simulink model "AOO_VOO_VVI_AAI_v4"  (R2025a)
settings: Solver=FixedStepAuto  StartTime=0.0  StopTime=10.0  FixedStep=1e-3  RelTol=1e-3  EnableMultiTasking=on
undefined symbols (not defined in the file or in its folder): D0, D1, D10, D11, D12, D13, D2, D3, D4, D5, D6, D7, D8, D9, PTA0, PTA1, PTA2, PTB23, PTB9, PTC16, PTC17, PTC2, PTC3, PTC4, PTD0, PTD1, PTD2, PTD3
libraries: frdmk64flib x16
settings Model: SimulationMode=external  ExtModeTrigDuration=5  Creator=emily  LastModifiedBy=tphil
settings SolverCC: AlgebraicLoopSolver=TrustRegion
settings OptimizationCC: EnhancedBackFolding=on  PassReuseOutputArgsAs=Individual arguments  ZeroExternalMemoryAtStartup=off  ZeroInternalMemoryAtStartup=off  MaxStackSize=64  OptimizeBlockOrder=speed  DifferentSizesBufferReuse=on  OptimizationCustomize=off  EfficientTunableParamExpr=on
settings DebuggingCC: ParameterTunabilityLossMsg=error  UnconnectedInputMsg=warning  UnconnectedOutputMsg=warning  UnconnectedLineMsg=warning
settings HardwareCC: ProdBitPerPointer=32.0  ProdBitPerSizeT=32.0  ProdBitPerPtrDiffT=32.0  ProdLargestAtomicInteger=Long  ProdLargestAtomicFloat=Double  ProdWordSize=32.0  ProdHWDeviceType=ARM Compatible->ARM Cortex
settings ModelReferenceCC: EnableRefExpFcnMdlSchedulingChecks=on
settings SFSimCC: MATLABDynamicMemAlloc=off
settings RTWCC: SystemTargetFile=ert.tlc  HardwareBoard=NXP FRDM-K64F  TLCOptions="-aInlineSetEventsForThisBaseRateFcn=TLC_FALSE -aSuppressMultiTaskScheduler=TLC_FALSE  -aRateBasedStepFcn=0"  TemplateMakefile=ert_default_tmf  Toolchain=GNU Tools for ARM Embedded Processors  GPUComputeCapability=3.5  Description=Embedded Coder
settings CodeAppCC: ForceParamTrailComments=on  IgnoreCustomStorageClasses=off  OperatorAnnotations=on  SimulinkDataObjDesc=on  SFDataObjDesc=on  InsertBlockDesc=on
settings ERTTargetCC: ExtModeTransport=0.0  ExtModeStaticAlloc=off  ExtModeMexFile=ext_comm  ExtModeIntrfLevel=Level1  InlinedParameterPlacement=Hierarchical  DynamicArrayContainerType=coder::array

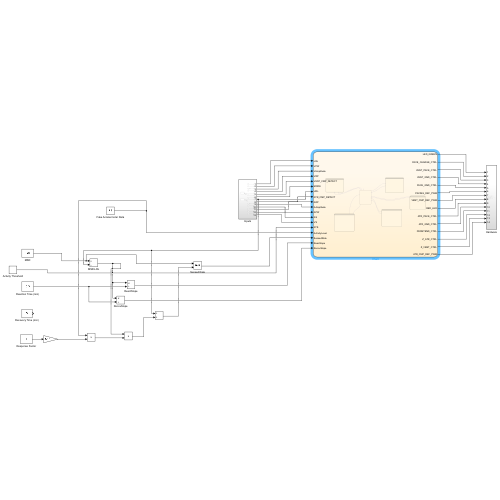
[thumbnail: Simulink's stored preview of the top-level diagram]
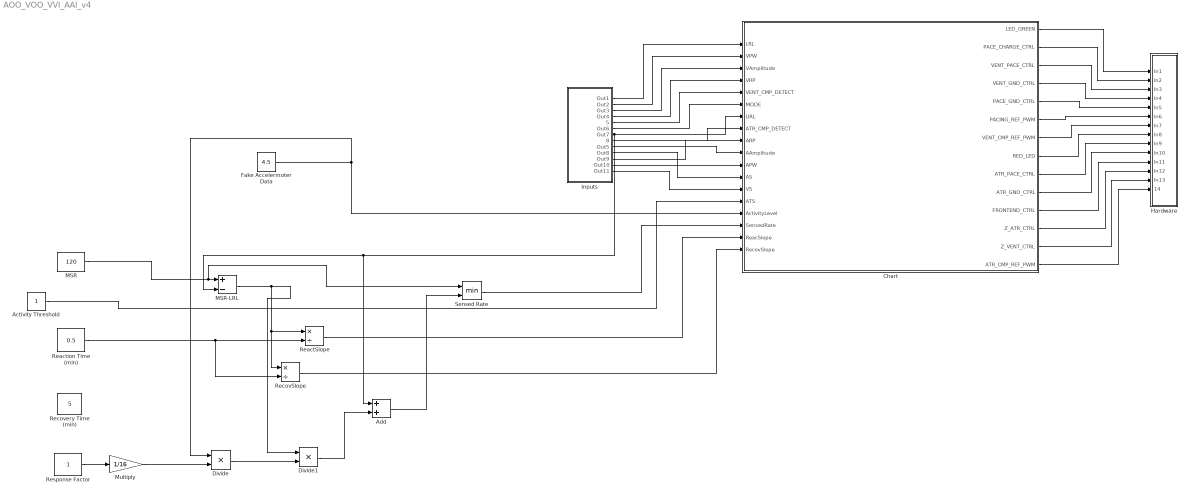
== system AOO_VOO_VVI_AAI_v4 ==
  Activity Threshold : Constant
  Add : Sum
  Chart : Stateflow chart  TreatAsAtomicUnit=on
  Divide : Product  Inputs=**
  Divide1 : Product  Inputs=**
  Fake Accelermoter Data : Constant  Value=4.5
  Hardware : Subsystem
  Inputs : Subsystem
  MSR : Constant  Value=120
  MSR-LRL : Sum  Inputs=+-
  Multiply : Gain  Gain=1/16
  ReactSlope : Product  Inputs=*/
  Reaction Time (min) : Constant  Value=0.5
  RecovSlope : Product  Inputs=*/
  Recovery Time (min) : Constant  Value=5
  Response Factor : Constant
  Sensed Rate : MinMax  Inputs=2
  wires:
  Chart/2(PACE_CHARGE_CTRL) -> Hardware/2(In2)
  Chart/4(VENT_GND_CTRL) -> Hardware/4(In4)
  Chart/12(Z_ATR_CTRL) -> Hardware/12(In12)
  Inputs/4(Out4) -> Chart/4(VRP)
  Chart/7(VENT_CMP_REF_PWM) -> Hardware/7(In7)
  Inputs/5(5) -> Chart/5(VENT_CMP_DETECT)
  Inputs/3(Out3) -> Chart/3(VAmplitude)
  Chart/3(VENT_PACE_CTRL) -> Hardware/3(In3)
  Inputs/6(Out6) -> Chart/6(MODE)
  Inputs/1(Out1) -> Chart/1(LRL)
  Chart/6(PACING_REF_PWM) -> Hardware/6(In6)
  Chart/13(Z_VENT_CTRL) -> Hardware/13(In13)
  Chart/9(ATR_PACE_CTRL) -> Hardware/9(In9)
  Chart/11(FRONTEND_CTRL) -> Hardware/11(In11)
  Chart/8(RED_LED) -> Hardware/8(In8)
  Chart/10(ATR_GND_CTRL) -> Hardware/10(In10)
  Inputs/2(Out2) -> Chart/2(VPW)
  Chart/5(PACE_GND_CTRL) -> Hardware/5(In5)
  Chart/1(LED_GREEN) -> Hardware/1(In1)
  Inputs/7(Out7) -> Add/1, MSR-LRL/2, Chart/7(URL)
  Inputs/8(8) -> Chart/8(ATR_CMP_DETECT)
  Chart/14(ATR_CMP_REF_PWM) -> Hardware/14(14)
  Inputs/9(Out5) -> Chart/10(AAmplitude)
  Inputs/10(Out8) -> Chart/11(APW)
  Inputs/11(Out9) -> Chart/9(ARP)
  Inputs/12(Out10) -> Chart/12(AS)
  Inputs/13(Out11) -> Chart/13(VS)
  MSR/1 -> Sensed Rate/1, MSR-LRL/1
  MSR-LRL/1 -> RecovSlope/1, ReactSlope/1, Divide1/1
  Reaction Time (min)/1 -> RecovSlope/2, ReactSlope/2
  Response Factor/1 -> Multiply/1
  Multiply/1 -> Divide/2
  Divide/1 -> Divide1/2
  Divide1/1 -> Add/2
  Add/1 -> Sensed Rate/2
  Sensed Rate/1 -> Chart/16(SensedRate)
  Activity Threshold/1 -> Chart/14(ATS)
  ReactSlope/1 -> Chart/17(ReacSlope)
  RecovSlope/1 -> Chart/18(RecovSlope)
  Fake Accelermoter Data/1 -> Divide/1, Chart/15(ActivityLevel)

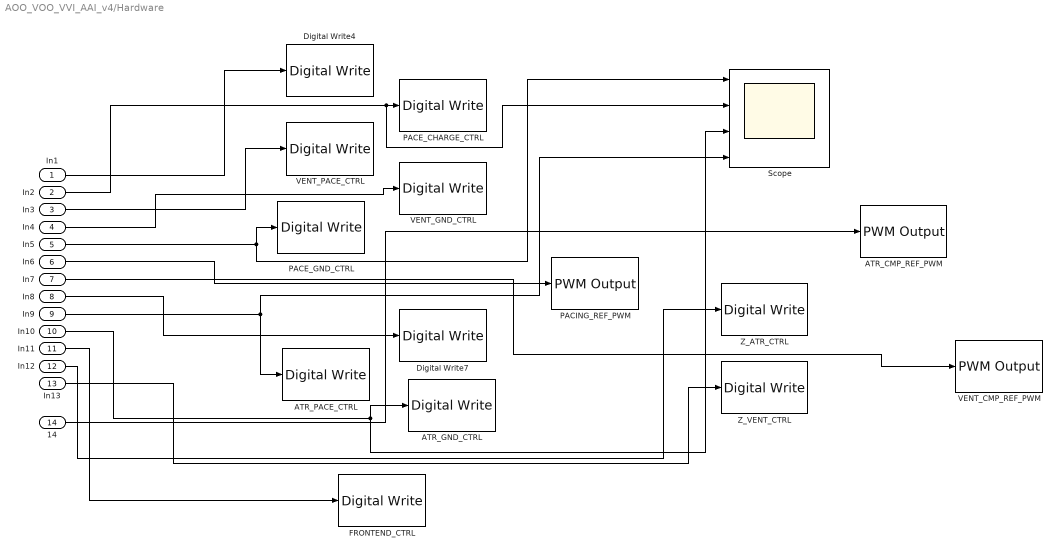
== system AOO_VOO_VVI_AAI_v4/Hardware ==
  In1 : Inport
  In2 : Inport  Port=2
  In3 : Inport  Port=3
  In4 : Inport  Port=4
  In5 : Inport  Port=5
  In6 : Inport  Port=6
  In7 : Inport  Port=7
  In8 : Inport  Port=8
  In9 : Inport  Port=9
  In10 : Inport  Port=10
  In11 : Inport  Port=11
  In12 : Inport  Port=12
  In13 : Inport  Port=13
  14 : Inport  Port=14
  ATR_CMP_REF_PWM : frdmk64flib/PWM Output  Whichpin=PTC2 (D6)  InitialFrequency=2000  InitialDutyCycle=0
  ATR_GND_CTRL : frdmk64flib/Digital Write  Whichpin=PTD2 (D11)
  ATR_PACE_CTRL : frdmk64flib/Digital Write  Whichpin=PTA0 (D8)
  Digital Write4 : frdmk64flib/Digital Write  Whichpin=GREEN_LED
  Digital Write7 : frdmk64flib/Digital Write  Whichpin=RED_LED
  FRONTEND_CTRL : frdmk64flib/Digital Write  Whichpin=PTD1 (D13)
  PACE_CHARGE_CTRL : frdmk64flib/Digital Write  Whichpin=PTB9 (D2)
  PACE_GND_CTRL : frdmk64flib/Digital Write  Whichpin=PTD0 (D10)
  PACING_REF_PWM : frdmk64flib/PWM Output  Whichpin=PTA2 (D5)  InitialFrequency=2000  InitialDutyCycle=30
  Scope : Scope  NumInputPorts=4
      settings: DataLoggingVariableName=ScopeData2
  VENT_CMP_REF_PWM : frdmk64flib/PWM Output  Whichpin=PTA1 (D3)  InitialFrequency=2000  InitialDutyCycle=0
  VENT_GND_CTRL : frdmk64flib/Digital Write  Whichpin=PTD3 (D12)
  VENT_PACE_CTRL : frdmk64flib/Digital Write  Whichpin=PTC4 (D9)
  Z_ATR_CTRL : frdmk64flib/Digital Write  Whichpin=PTB23 (D4)
  Z_VENT_CTRL : frdmk64flib/Digital Write  Whichpin=PTC3 (D7)
  wires:
  In10/1 -> Scope/3, ATR_GND_CTRL/1
  In2/1 -> Scope/2, PACE_CHARGE_CTRL/1
  In6/1 -> PACING_REF_PWM/1
  In4/1 -> VENT_GND_CTRL/1
  In13/1 -> Z_VENT_CTRL/1
  In1/1 -> Digital Write4/1
  In5/1 -> PACE_GND_CTRL/1, Scope/1
  In3/1 -> VENT_PACE_CTRL/1
  In9/1 -> ATR_PACE_CTRL/1, Scope/4
  In8/1 -> Digital Write7/1
  In12/1 -> Z_ATR_CTRL/1
  In11/1 -> FRONTEND_CTRL/1
  14/1 -> ATR_CMP_REF_PWM/1
  In7/1 -> VENT_CMP_REF_PWM/1

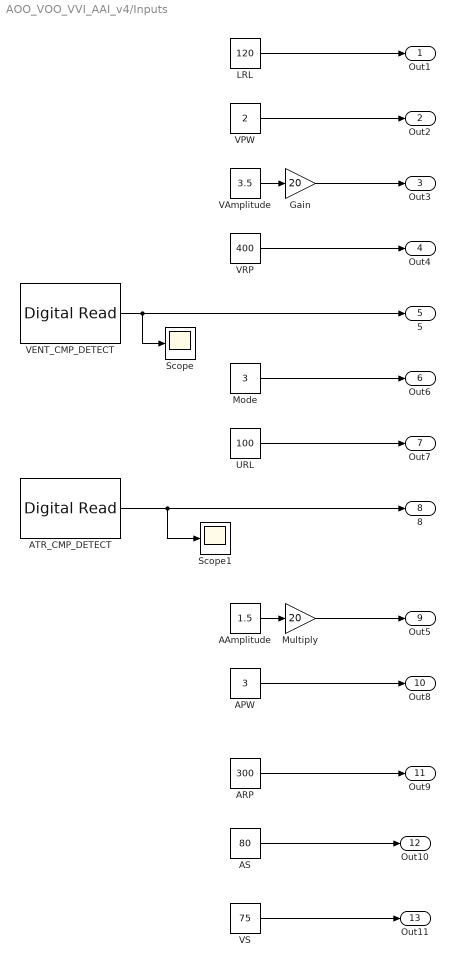
== system AOO_VOO_VVI_AAI_v4/Inputs ==
  AAmplitude : Constant  Value=1.5  OutDataTypeStr=double
  APW : Constant  Value=3  OutDataTypeStr=double
  ARP : Constant  Value=300  OutDataTypeStr=double
  AS : Constant  Value=80  OutDataTypeStr=double
  ATR_CMP_DETECT : frdmk64flib/Digital Read  Whichpin=PTC16 (D0)  SampleTime=-1
  Gain : Gain  Gain=20
  LRL : Constant  Value=120  OutDataTypeStr=double
  Mode : Constant  Value=3  OutDataTypeStr=int16
  Multiply : Gain  Gain=20
  Scope : Scope
      settings: ActiveDisplayYMinimum=0.9  ActiveDisplayYMaximum=1.1
  Scope1 : Scope
      settings: ActiveDisplayYMinimum=0.9  ActiveDisplayYMaximum=1.1
  URL : Constant  Value=100  OutDataTypeStr=double
  VAmplitude : Constant  Value=3.5  OutDataTypeStr=double
  VENT_CMP_DETECT : frdmk64flib/Digital Read  Whichpin=PTC17 (D1)  SampleTime=inf
  VPW : Constant  Value=2  OutDataTypeStr=double
  VRP : Constant  Value=400  OutDataTypeStr=double
  VS : Constant  Value=75  OutDataTypeStr=double
  Out1 : Outport
  Out2 : Outport  Port=2
  Out3 : Outport  Port=3
  Out4 : Outport  Port=4
  5 : Outport  Port=5
  Out6 : Outport  Port=6
  Out7 : Outport  Port=7
  8 : Outport  Port=8
  Out5 : Outport  Port=9
  Out8 : Outport  Port=10
  Out9 : Outport  Port=11
  Out10 : Outport  Port=12
  Out11 : Outport  Port=13
  wires:
  VPW/1 -> Out2/1
  VAmplitude/1 -> Gain/1
  VENT_CMP_DETECT/1 -> 5/1, Scope/1
  VRP/1 -> Out4/1
  Mode/1 -> Out6/1
  LRL/1 -> Out1/1
  Gain/1 -> Out3/1
  URL/1 -> Out7/1
  ATR_CMP_DETECT/1 -> Scope1/1, 8/1
  AAmplitude/1 -> Multiply/1
  Multiply/1 -> Out5/1
  APW/1 -> Out8/1
  ARP/1 -> Out9/1
  AS/1 -> Out10/1
  VS/1 -> Out11/1

== stateflow chart AOO_VOO_VVI_AAI_v4/Chart ==
  state VOO
    entry:
    % Initialize PACE_GND_CTRL and set the PWM amplitude to the Ventricular Amplitude
    PACE_GND_CTRL = 1;
    PACING_REF_PWM = VAmplitude;
    state TIMING
      entry:
      % upon entry into VOO send no pulse
      % and wait for a period - the VPW
      LED_GREEN = 0;
      VENT_PACE_CTRL = 0;
      PACE_CHARGE_CTRL =1;
      VENT_GND_CTRL = 1;
    state PULSE
      entry:
      % upon entry into VOO send no pulse
      % and wait for a period - the VPW
      LED_GREEN = 1;
      PACE_CHARGE_CTRL =0;
      VENT_PACE_CTRL = 1;
      VENT_GND_CTRL = 0;
    (default) -> VOO.TIMING
    VOO.PULSE -> VOO.TIMING : after(VPW, msec)
    VOO.TIMING -> VOO.PULSE : after(60000/LRL -VPW, msec)
  state AOO
    entry:
    % Initialize PACE_GND_CTRL and set the PWM amplitude to the Atrial Amplitude
    PACE_GND_CTRL = 1;
    PACING_REF_PWM = VAmplitude;
    state TIMING
      entry:
      % upon entry into AOO send no pulse
      % and wait for a period - the APW
      LED_GREEN = 0;
      ATR_PACE_CTRL = 0;
      PACE_CHARGE_CTRL =1;
      ATR_GND_CTRL = 1;
    state PULSE
      entry:
      % after set duration has passed, send
      % a pulse for the APW duration
      LED_GREEN = 1;
      PACE_CHARGE_CTRL =0;
      ATR_GND_CTRL = 0;
      ATR_PACE_CTRL = 1;
    (default) -> AOO.TIMING
    AOO.TIMING -> AOO.PULSE : after(60000/LRL -APW, msec)
    AOO.PULSE -> AOO.TIMING : after(APW, msec)
  state INITIALIZE
    entry:
    % Initialize inputs
    PACE_CHARGE_CTRL = 0;
    ATR_PACE_CTRL = 0;
    VENT_PACE_CTRL = 0;
    PACE_GND_CTRL = 1;
    ATR_GND_CTRL = 0;
    VENT_GND_CTRL=0;
    FRONTEND_CTRL=1;
    Z_ATR_CTRL = 0;
    Z_VENT_CTRL=0;
  state VVIR
    entry:
    % set PACE_GND_CTRL to 1 and the PWM amplitude to Ventricular Amplitude
    PACE_GND_CTRL = 1;
    PACING_REF_PWM = VAmplitude;
    % Set the ATR_CMP_REF_PWM to Ventricular sensitivity
    VENT_CMP_REF_PWM=VS;
    HeartRate = LRL
    %actTime and noactTime needs to be in mins
    actTime = 0
    noactTime = 0
    state AtSensedRate
      entry:
      HeartRate = SensedRate
    state IncreaseHeartRate
      entry:
      HeartRate = HeartRate+ReacSlope*actTime
    state WAIT
      entry:
      entry:
      % upon entry wait for signal to be
      % sensed or duration of no pulse
      % to pass
      PACE_CHARGE_CTRL = 1;
      Z_VENT_CTRL=1;
      VENT_PACE_CTRL = 0;
      VENT_GND_CTRL =1;
      RED_LED = 0;
      LED_GREEN = 0;
    state DecreaseHeartRate
      entry:
      HeartRate=HeartRate-RecovSlope*noactTime
    state AtLRL
      entry:
      HeartRate = LRL
    state PACE
      entry:
      % if no signal was sensed send pulse
      PACE_CHARGE_CTRL = 0;
      Z_VENT_CTRL=0;
      VENT_PACE_CTRL = 1;
      VENT_GND_CTRL = 0;
      RED_LED = 0;
      LED_GREEN = 1;
    state REFRACTORY
      entry:
      % if signal was sensed or VPW duration passed
      % wait for VRP duration and go to WAIT state
      PACE_CHARGE_CTRL = 1;
      Z_VENT_CTRL=1;
      VENT_PACE_CTRL = 0;
      VENT_GND_CTRL = 1;
      RED_LED = 1;
      LED_GREEN = 0;
    AtSensedRate -> (junction 162)
    (junction 143) -> AtSensedRate [order 1] : [HeartRate+ReacSlope*actTime>=SensedRate]
    (default) -> VVIR.WAIT
    VVIR.WAIT -> (junction 143) [order 2] : [ActivityLevel - ATS > 0]
    (junction 143) -> IncreaseHeartRate [order 2] : [HeartRate+ReacSlope*actTime < SensedRate]
    IncreaseHeartRate -> (junction 162)
    (junction 162) -> VVIR.WAIT
    AtLRL -> (junction 162)
    DecreaseHeartRate -> (junction 162)
    VVIR.WAIT -> (junction 150) [order 4] : [ActivityLevel - ATS < 0]
    (junction 150) -> DecreaseHeartRate [order 1] : [HeartRate-RecovSlope*noactTime > LRL]
    (junction 150) -> AtLRL [order 2] : [HeartRate-RecovSlope*noactTime <= LRL]
    VVIR.WAIT -> VVIR.REFRACTORY [order 1] : [VENT_CMP_DETECT == 1]
    VVIR.REFRACTORY -> VVIR.WAIT : after(VRP,msec)
    VVIR.WAIT -> VVIR.PACE [order 3] : after(60000/HeartRate - (VPW+VRP), msec)
    VVIR.PACE -> VVIR.REFRACTORY : after(VPW, msec)
  state VVI
    entry:
    % set PACE_GND_CTRL to 1 and the PWM amplitude to Ventricular Amplitude
    PACE_GND_CTRL = 1;
    PACING_REF_PWM = VAmplitude;
    % Set the ATR_CMP_REF_PWM to Ventricular sensitivity
    VENT_CMP_REF_PWM=VS;
    state PACE
      entry:
      % if no signal was sensed send pulse
      PACE_CHARGE_CTRL = 0;
      Z_VENT_CTRL=0;
      VENT_PACE_CTRL = 1;
      VENT_GND_CTRL = 0;
      RED_LED = 0;
      LED_GREEN = 1;
    state WAIT
      entry:
      % upon entry wait for signal to be
      % sensed or duration of no pulse
      % to pass
      PACE_CHARGE_CTRL = 1;
      Z_VENT_CTRL=1;
      VENT_PACE_CTRL = 0;
      VENT_GND_CTRL =1;
      RED_LED = 0;
      LED_GREEN = 0;
    state REFRACTORY
      entry:
      % if signal was sensed or VPW duration passed
      % wait for VRP duration and go to WAIT state
      PACE_CHARGE_CTRL = 1;
      Z_VENT_CTRL=1;
      VENT_PACE_CTRL = 0;
      VENT_GND_CTRL = 1;
      RED_LED = 1;
      LED_GREEN = 0;
    (default) -> VVI.WAIT
    VVI.WAIT -> VVI.PACE [order 1] : after(60000/LRL -(VPW+VRP), msec)
    VVI.PACE -> VVI.REFRACTORY : after(VPW,msec)
    VVI.WAIT -> VVI.REFRACTORY [order 2] : [VENT_CMP_DETECT==1]
    VVI.REFRACTORY -> VVI.WAIT : after(VRP, msec)
  state AAI
    entry:
    % set PACE_GND_CTRL to 1 and the PWM amplitude to Atrial Amplitude
    PACE_GND_CTRL = 1;
    PACING_REF_PWM = AAmplitude;
    % Set the ATR_CMP_REF_PWM to Atrial sensitivity
    ATR_CMP_REF_PWM=AS;
    state PACE
      entry:
      % if no signal was sensed send pulse
      PACE_CHARGE_CTRL = 0;
      ATR_PACE_CTRL = 1;
      ATR_GND_CTRL = 0;
      RED_LED = 0;
      LED_GREEN = 1;
    state WAIT
      entry:
      % upon entry wait for signal to be
      % sensed or duration of no pulse
      % to pass
      PACE_CHARGE_CTRL = 1;
      ATR_PACE_CTRL = 0;
      ATR_GND_CTRL =1;
      RED_LED = 0;
      LED_GREEN = 0;
    state REFRACTORY
      entry:
      % if signal was sensed or APW duration passed
      % wait for ARP duration and go to WAIT state
      PACE_CHARGE_CTRL = 1;
      ATR_PACE_CTRL = 0;
      ATR_GND_CTRL = 1;
      RED_LED = 1;
      LED_GREEN = 0;
    (default) -> AAI.WAIT
    AAI.WAIT -> AAI.PACE [order 1] : after(60000/LRL -(APW+ARP), msec)
    AAI.WAIT -> AAI.REFRACTORY [order 2] : [ATR_CMP_DETECT==1]
    AAI.REFRACTORY -> AAI.WAIT : after(ARP, msec)
    AAI.PACE -> AAI.REFRACTORY : after(APW,msec)
  INITIALIZE -> VOO [order 2] : [MODE==2]
  VOO -> INITIALIZE : [MODE~=2]
  AOO -> INITIALIZE : [MODE~=1]
  INITIALIZE -> AOO [order 1] : [MODE==1]
  (default) -> INITIALIZE
  AAI -> INITIALIZE : [MODE~=4]
  INITIALIZE -> VVIR [order 3] : [MODE==5]
  VVIR -> INITIALIZE : [MODE~=5]
  INITIALIZE -> VVI [order 5] : [MODE==3]
  VVI -> INITIALIZE : [MODE~=3]
  INITIALIZE -> AAI [order 4] : [MODE==4]
  data: LRL input double; VPW input double; LED_GREEN output int16; PACE_CHARGE_CTRL output int16; VENT_PACE_CTRL output int16; VENT_GND_CTRL output int16; PACE_GND_CTRL output int16; PACING_REF_PWM output double; VAmplitude input double; VRP input double; VENT_CMP_DETECT input boolean; MODE input int16; VENT_CMP_REF_PWM output; RED_LED output; ATR_PACE_CTRL output; ATR_GND_CTRL output; FRONTEND_CTRL output; Z_ATR_CTRL output; Z_VENT_CTRL output; URL input; ATR_CMP_DETECT input; ATR_CMP_REF_PWM output; ARP input double; AAmplitude input double; APW input double; AS input double; VS input double; ATS input double; ActivityLevel input; SensedRate input double; ReacSlope input; RecovSlope input; HeartRate local; actTime local double; noactTime local double
